simulink model "MRFMDOB"  (R2016b)
settings: Solver=ode45  StartTime=0.0  StopTime=5  FixedStep=Tu/10  MaxStep=Tu/10  RelTol=1e-3  EnableMultiTasking=on
values from neighbouring files (symbols this model uses):
  L = 4    [FIR_MMP_example.m]    (also in IIR_MMP_example.m; MMP_prediction_general.m = 6; MMP_simulink.m; MMPexample.m)
  PRpara = MMP(Apara,L)    [mainMRDOB.m]
  Ts = 0.0008    [mainIIR_MMP.m]    (also in mainMRDOB.m = 0.005)
  Tu = Ts/L    [IIR_MMP.m]    (also in MMPexample.m = 0.4; mainIIR_MMP.m = 0.0004; mainMRDOB.m = 0.0025)
undefined symbols (not defined in the file or in its folder): dist
libraries: cstblocks x3, dspsigops x1
settings Model: Creator=hux15002  LastModifiedBy=Hui Xiao
settings DataIOCC: LimitDataPoints=on
settings OptimizationCC: LifeSpan=inf
settings DebuggingCC: AllowSymbolicDim=off  SFUnexpectedBacktrackingDiag=warning  SFNoUnconditionalDefaultTransitionDiag=warning  SFExecutionAtInitializationDiag=none
settings ModelReferenceCC: PropagateSignalLabelsOutOfModel=off
settings GRTTargetCC: TargetLangStandard=C89/C90 (ANSI)
settings ConfigComp: CovMetricSettings=dw  CovHtmlReporting=on  CovSaveCumulativeToWorkspaceVar=on  CovSaveSingleToWorkspaceVar=on  CovExternalEMLEnable=off

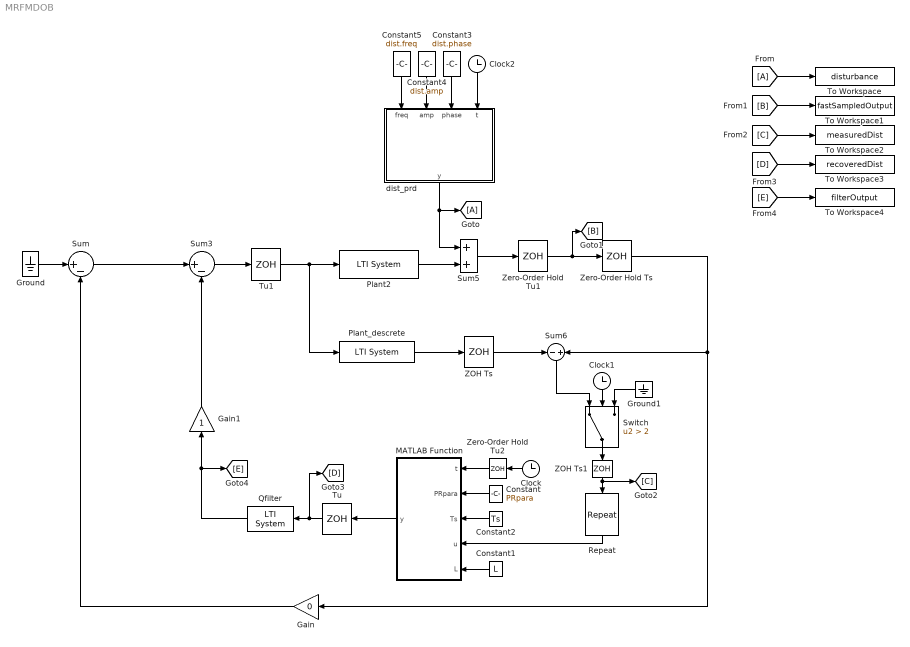
== system MRFMDOB ==
  " dist_prd" : MATLAB Function  TreatAsAtomicUnit=on
  Clock : Clock
  Clock1 : Clock
  Clock2 : Clock
  Constant : Constant  Value=PRpara  VectorParams1D=off
  Constant1 : Constant  Value=L
  Constant2 : Constant  Value=Ts
  Constant3 : Constant  Value=dist.phase
  Constant4 : Constant  Value=dist.amp
  Constant5 : Constant  Value=dist.freq
  Gain : Gain  Gain=0
  Gain1 : Gain
  Ground : Ground
  Ground1 : Ground
  MATLAB Function : MATLAB Function  TreatAsAtomicUnit=on
  Plant2 : cstblocks/LTI System  sys=PdL  IC=0
  Plant_descrete : cstblocks/LTI System  sys=PdL  IC=[]
  Qfilter : cstblocks/LTI System  sys=QFM  IC=[]
  Repeat : dspsigops/Repeat  N=L  RateOptions=Allow multirate processing  ic=0  mode=Unused parameter value
  Sum : Sum  Inputs=|+-  SaturateOnIntegerOverflow=on
  Sum3 : Sum  Inputs=|+-
  Sum5 : Sum  SaturateOnIntegerOverflow=on
  Sum6 : Sum  Inputs=-|+
  Switch : Switch  Criteria=u2 > Threshold  Threshold=2
  To Workspace : ToWorkspace  VariableName=disturbance  SaveFormat=Structure With Time  SampleTime=-1
  To Workspace1 : ToWorkspace  VariableName=fastSampledOutput  SaveFormat=Structure With Time  SampleTime=-1
  To Workspace2 : ToWorkspace  VariableName=measuredDist  SaveFormat=Structure With Time  SampleTime=-1
  To Workspace3 : ToWorkspace  VariableName=recoveredDist  SaveFormat=Structure With Time  SampleTime=-1
  To Workspace4 : ToWorkspace  VariableName=filterOutput  SaveFormat=Structure With Time  SampleTime=-1
  Tu : ZeroOrderHold  SampleTime=Tu
  Tu1 : ZeroOrderHold  SampleTime=Tu
  ZOH Ts : ZeroOrderHold  SampleTime=Ts
  ZOH Ts1 : ZeroOrderHold  SampleTime=Ts
  Zero-Order Hold Ts : ZeroOrderHold  SampleTime=Ts
  Zero-Order Hold Tu1 : ZeroOrderHold  SampleTime=Tu
  Zero-Order Hold Tu2 : ZeroOrderHold  SampleTime=Tu
  wires:
  Ground/1 -> Sum/1
  Zero-Order Hold Ts/1 -> Sum6/2, Gain/1
  Sum3/1 -> Tu1/1
  Constant/1 -> MATLAB Function/2(PRpara)
  Constant2/1 -> MATLAB Function/3(Ts)
  Sum5/1 -> Zero-Order Hold Tu1/1
  MATLAB Function/1(y) -> Tu/1
  Plant_descrete/1 -> ZOH Ts/1
  ZOH Ts/1 -> Sum6/1
  Tu1/1 -> Plant_descrete/1, Plant2/1
  Tu/1 -> [D], Qfilter/1
  Sum/1 -> Sum3/1
  Plant2/1 -> Sum5/2
  " dist_prd"/1(y) -> [A], Sum5/1
  Qfilter/1 -> [E], Gain1/1
  Zero-Order Hold Tu1/1 -> [B], Zero-Order Hold Ts/1
  Repeat/1 -> MATLAB Function/4(u)
  Clock1/1 -> Switch/2
  Switch/1 -> ZOH Ts1/1
  ZOH Ts1/1 -> [C], Repeat/1
  Sum6/1 -> Switch/1
  Ground1/1 -> Switch/3
  Zero-Order Hold Tu2/1 -> MATLAB Function/1(t)
  Clock/1 -> Zero-Order Hold Tu2/1
  Clock2/1 -> " dist_prd"/4(t)
  Constant5/1 -> " dist_prd"/1(freq)
  Constant4/1 -> " dist_prd"/2(amp)
  Constant3/1 -> " dist_prd"/3(phase)
  Constant1/1 -> MATLAB Function/5(L)
  Gain/1 -> Sum/2
  Gain1/1 -> Sum3/2
  [A] -> To Workspace/1
  [B] -> To Workspace1/1
  [C] -> To Workspace2/1
  [E] -> To Workspace4/1
  [D] -> To Workspace3/1

== matlab function MRFMDOB/ dist_prd ==
  settings: updateMethod=CONTINUOUS
  data: freq input; y output; amp input; phase input; t input
function y = dist_prd(freq,amp,phase,t)
y = 0;
for i=1:length(freq)
    y = y + amp(i)*sin(2*pi*freq(i)*t+phase(i));
end
end

== matlab function MRFMDOB/MATLAB Function ==
  settings: updateMethod=DISCRETE  sampleTime=Tu
  data: t input; PRpara input; Ts input; u input; y output; L input
function y = MRIMP(t, PRpara, Ts, u, L)
% Hui Xiao 10-14-2016
persistent phi;
persistent ylast;
persistent tlast;
[~,m] = size(PRpara);
if isempty(phi)
    phi = zeros(m,1);
    tlast = t;
    ylast = 0;
end

%if this function is called at a same time multiple times,
%just update the phi table once.
if t == tlast
    y = ylast;
    return
end
tlast = t;

Tu = Ts/L;
if (mod(t,Ts) > -Tu/10) && (mod(t,Ts) < Tu/10)
    %update phi
    for i=m:-1:2
        phi(i)=phi(i-1);
    end
    phi(1)=u;
    %disp(t)
    %disp(phi)
    y = u;
    ylast = y;
else
    index = round(mod(t,Ts)/Tu);
    y = 0;
    for i = 1:m
        y=y+PRpara(index,i)*phi(i);
        %disp(index)
    end
    ylast = y;
end
end
